simulink model "ex_04_04"  (R2024a)
settings: Solver=VariableStepAuto  StartTime=0.0  StopTime=10  MaxStep=0.001  RelTol=1e-3
settings Model: Creator=vpetrone  LastModifiedBy=vpetrone
settings ModelReferenceCC: EnableRefExpFcnMdlSchedulingChecks=on
settings RTWCC: GPUComputeCapability=3.5

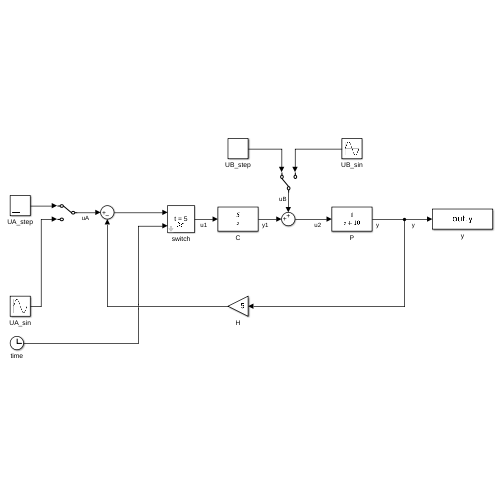
[thumbnail: Simulink's stored preview of the top-level diagram]
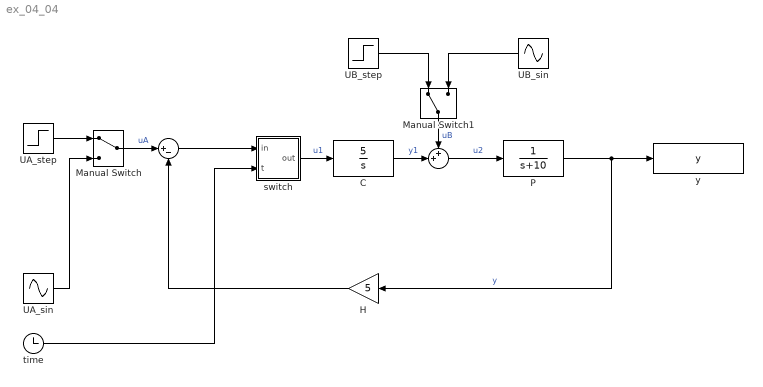
== system ex_04_04 ==
  " " : Sum  Inputs=++|
  "   " : Sum  Inputs=|+-
  C : TransferFcn  Numerator=[5]  Denominator=[1 0]
  H : Gain  Gain=5
  Manual Switch : ManualSwitch
  Manual Switch1 : ManualSwitch
  P : TransferFcn  Denominator=[1 10]
  UA_sin : Sin  Frequency=0.1  SampleTime=0
  UA_step : Step  Time=0  After=10  SampleTime=0
  UB_sin : Sin  Frequency=10  SampleTime=0
  UB_step : Step  Time=3  After=2  SampleTime=0
  switch : Subsystem  mask{T=5}
      mask prompts: T "opening_time"
      mask Display:
      | image('assets/switch.png'); % Use "Edit Image" on toolstrip to change.
      | TT = get_param(gcb, 'opening_time');
      | disp(['t = ' TT])
  time : Clock
  y : ToWorkspace  VariableName=y  SaveFormat=Timeseries  SampleTime=-1
  wires:
  UA_step/1 -> Manual Switch/1
  UA_sin/1 -> Manual Switch/2
  switch/1(out) -> C/1  "u1"
  time/1 -> switch/2(t)
  UB_sin/1 -> Manual Switch1/2
  UB_step/1 -> Manual Switch1/1
  Manual Switch/1 -> "   "/1  "uA"
  H/1 -> "   "/2
  "   "/1 -> switch/1(in)
  " "/1 -> P/1  "u2"
  P/1 -> H/1, y/1  "y"
  C/1 -> " "/2  "y1"
  Manual Switch1/1 -> " "/1  "uB"

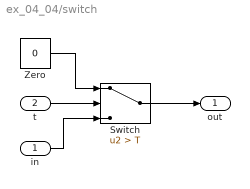
== system ex_04_04/switch ==
  in : Inport
  t : Inport  Port=2
  Switch : Switch  Criteria=u2 > Threshold  Threshold=T  SaturateOnIntegerOverflow=off  InputSameDT=off
  Zero : Constant  Value=0  OutDataTypeStr=Inherit: Inherit via back propagation
  out : Outport
  wires:
  t/1 -> Switch/2
  in/1 -> Switch/3
  Switch/1 -> out/1
  Zero/1 -> Switch/1
